simulink model "UnitTestDebug"  (R2018b)
settings: Solver=FixedStepAuto  StartTime=0.0  StopTime=500  FixedStep=fswParams.sample_time_s  RelTol=1e-3
undefined symbols (not defined in the file): DiscIntNeverNeededParam, fswParams, MEKF_lib, simParams, Triad, Triad_lib
libraries: aerolibutil x7, simulink x6, vrlib x4, sharedutil x3, sharedtransform x3, dspmathops x2, satelliteDynamics_lib x1
(part 1 of 2)
settings Model: SimulationMode=accelerator  Creator=satcave1  LastModifiedBy=kylle
settings OptimizationCC: EfficientMapNaN2IntZero=off
settings HardwareCC: TargetBitPerPointer=64  TargetBitPerSizeT=64  TargetBitPerPtrDiffT=64  TargetLongLongMode=on  TargetIntDivRoundTo=Zero  TargetEndianess=LittleEndian  TargetWordSize=64  TargetHWDeviceType=MATLAB Host  ProdEqTarget=off
settings CodeAppCC: MaxIdLength=128
settings GRTTargetCC: TargetLangStandard=C89/C90 (ANSI)  CombineOutputUpdateFcns=off  GRTInterface=on

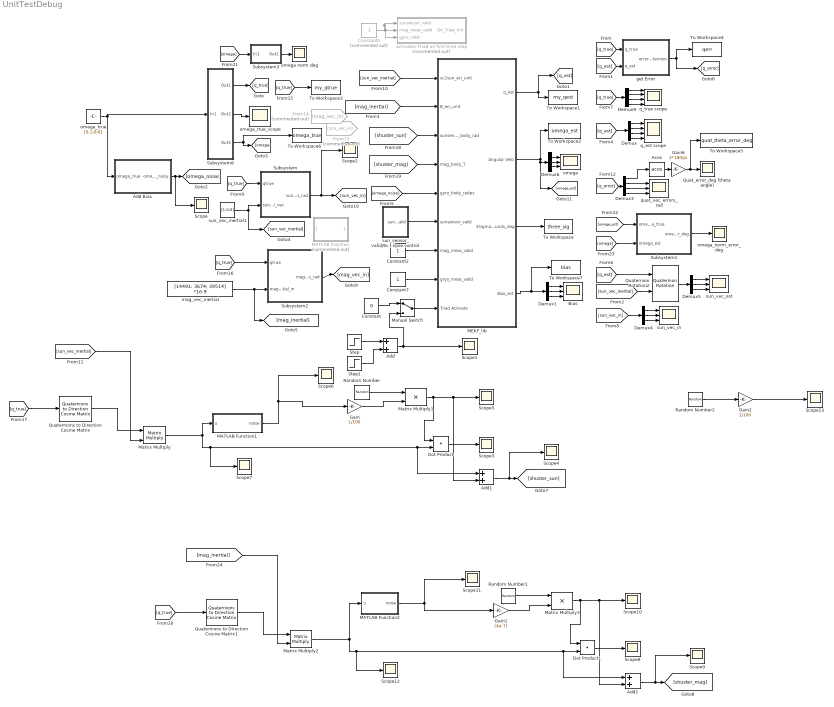
== system UnitTestDebug ==
  Acos : Trigonometry  Operator=acos
  Add : Sum
  Add Bias : Subsystem
  Add1 : Sum
  Add2 : Sum
  Bias : Scope  NumInputPorts=3
  Constant : Constant  Value=0
  Constant2 : Constant
  Constant5 : Constant  Commented=on
  Constant7 : Constant
  Demux : Demux
  Demux{1,4..6} (4 alike) : Demux  Outputs=3
  Demux3 : Demux
  Demux9 : Demux
  Dot Product : DotProduct  InputSameDT=on  OutDataTypeStr=Inherit: Inherit via internal rule
  Dot Product1 : DotProduct  InputSameDT=on  OutDataTypeStr=Inherit: Inherit via internal rule
  From13 : From  Commented=on  GotoTag=sun_vec_in
  From14 : From  Commented=on  GotoTag=mag_vec_in
  Gain : Gain  Gain=1/100
  Gain1 : Gain  Gain=(4e-7)
  Gain2 : Gain  Gain=1/100
  Gain6 : Gain  Gain=2*180/pi
  MATLAB Function : MATLAB Function  Commented=on  TreatAsAtomicUnit=on
  MATLAB Function1 : MATLAB Function  TreatAsAtomicUnit=on
  MATLAB Function2 : MATLAB Function  TreatAsAtomicUnit=on
  MEKF_lib : Subsystem  AncestorBlock=MEKF_lib/MEKF_lib
  Manual Switch : ManualSwitch
  Matrix Multiply : Product  Multiplication=Matrix(*)
  Matrix Multiply1 : Product
  Matrix Multiply2 : Product  Multiplication=Matrix(*)
  Matrix Multiply3 : Product
  Quat_error_deg (theta angle) : Scope
  Quaternion Rotation2 : aerolibutil/Quaternion Rotation
  Quaternions to Direction Cosine Matrix : sharedtransform/Quaternions to  Direction Cosine Matrix  aMode=aMode
      settings: SourceProductName=Aerospace Blockset  SourceProductBaseCode=AE
  Quaternions to Direction Cosine Matrix1 : sharedtransform/Quaternions to  Direction Cosine Matrix  aMode=aMode
      settings: SourceProductName=Aerospace Blockset  SourceProductBaseCode=AE
  Random Number : RandomNumber  Variance=[1;1;1]  SampleTime=0.1
  Random Number1 : RandomNumber  Variance=[1;1;1]  SampleTime=0.1
  Random Number2 : RandomNumber  Variance=[1;1;1]  SampleTime=0.1
  Scope{,1..13} (14 alike) : Scope
  Step : Step  Time=300  SampleTime=0
  Step1 : Step  Time=fswParams.sample_time_s+340  After=-1  SampleTime=0
  Subsystem : Subsystem
  Subsystem1 : Subsystem
  Subsystem2 : Subsystem
  Subsystem3 : Subsystem
  Subsystem8 : Subsystem
  To Workspace : ToWorkspace  VariableName=three_sig  SaveFormat=Structure With Time  SampleTime=-1
  To Workspace1 : ToWorkspace  VariableName=my_qest  SaveFormat=Structure With Time  SampleTime=-1
  To Workspace2 : ToWorkspace  VariableName=omega_est  SaveFormat=Structure  SampleTime=-1
  To Workspace3 : ToWorkspace  VariableName=my_qtrue  SaveFormat=Structure With Time  SampleTime=-1
  To Workspace4 : ToWorkspace  VariableName=qerr  SaveFormat=Structure With Time  SampleTime=-1
  To Workspace5 : ToWorkspace  VariableName=quat_theta_error_deg  SaveFormat=Structure With Time  SampleTime=-1
  To Workspace6 : ToWorkspace  VariableName=omega_true  SaveFormat=Structure  SampleTime=-1
  To Workspace7 : ToWorkspace  VariableName=bias  SaveFormat=Structure With Time  SampleTime=-1
  "activates Triad on first time step " : Subsystem  Commented=on
  get Error : Subsystem
  mag_vec_inertial : Constant  Value=[14491; 3674; 39514] *1e-9  VectorParams1D=off
  omega : Scope  NumInputPorts=3
  omega norm deg : Scope
  omega_norm_error_deg : Scope
  omega_true : Constant  Value=[0.1;0;0]  VectorParams1D=off
  omega_true_scope : Scope
  q_est scope : Scope  NumInputPorts=4
  "q_true scope " : Scope  NumInputPorts=4
  quat_vec_errors_rad : Scope  NumInputPorts=3
  sun_sensor_valid/Eclipse control : Subsystem
  sun_vec_est : Scope  NumInputPorts=3
  sun_vec_in : Scope  NumInputPorts=3
  sun_vec_inertial1 : Constant  Value=[1;0;0]  VectorParams1D=off
  wires:
  Demux/2 -> q_est scope/2
  Demux/3 -> q_est scope/3
  Demux/4 -> q_est scope/4
  Demux1/2 -> Bias/2
  Demux1/1 -> Bias/1
  Demux1/3 -> Bias/3
  Constant7/1 -> MEKF_lib/8(gryo_meas_valid)
  [sun_vec_inertial] -> MEKF_lib/1(sc2sun_eci_unit)
  [mag_inertial] -> MEKF_lib/2(B_eci_unit)
  MEKF_lib/3("3Sigma Bounds_deg ") -> To Workspace/1
  MEKF_lib/4(Bias_est) -> To Workspace7/1, Demux1/1
  MEKF_lib/1(q_est) -> To Workspace1/1, [q_est]
  [omega_noise] -> MEKF_lib/5(gyro_body_radps)
  Demux4/1 -> sun_vec_in/1
  Demux4/3 -> sun_vec_in/3
  Demux4/2 -> sun_vec_in/2
  [sun_vec_inertial] -> Quaternion Rotation2/2
  [q_est] -> Quaternion Rotation2/1
  Quaternion Rotation2/1 -> Demux5/1
  Demux5/1 -> sun_vec_est/1
  Demux5/2 -> sun_vec_est/2
  Demux6/1 -> omega/1
  Demux6/3 -> omega/3
  MEKF_lib/2("Angular Velo ") -> [omege_est], Demux6/1, To Workspace2/1
  Add/1 -> Manual Switch/2, Scope1/1
  Constant5/1 -> "activates Triad on first time step "/1(sunsensor_valid), "activates Triad on first time step "/3(gyro_valid), "activates Triad on first time step "/2(mag_meas_valid)
  Demux5/3 -> sun_vec_est/3
  Demux3/2 -> quat_vec_errors_rad/1
  Demux3/4 -> quat_vec_errors_rad/3
  [q_true] -> Demux9/1
  [q_true] -> get Error/1(q_true)
  [q_est] -> get Error/2(q_est)
  [sun_vec_in] -> Demux4/1
  [q_true] -> To Workspace3/1
  [q_est] -> Demux/1
  Demux/1 -> q_est scope/1
  Demux9/4 -> "q_true scope "/4
  Demux9/3 -> "q_true scope "/3
  Demux9/2 -> "q_true scope "/2
  Demux9/1 -> "q_true scope "/1
  Demux3/3 -> quat_vec_errors_rad/2
  get Error/1(error_quaternion) -> To Workspace4/1, [q_error]
  Constant2/1 -> MEKF_lib/7(mag_meas_valid)
  Demux3/1 -> Acos/1
  Acos/1 -> Gain6/1
  Gain6/1 -> To Workspace5/1, Quat_error_deg (theta angle)/1
  Subsystem8/1(Out1) -> [q_true]
  Subsystem8/2(Out2) -> omega_true_scope/1
  Subsystem8/3(Out5) -> [omega], To Workspace6/1
  [omege_est] -> Subsystem1/1(omega_true)
  [omega] -> Subsystem1/2(omega_est)
  Subsystem1/1(omega_norm_error_deg) -> omega_norm_error_deg/1
  [q_error] -> Demux3/1
  sun_sensor_valid/Eclipse control/1(sun_valid) -> MEKF_lib/6(sunsensor_valid)
  Demux6/2 -> omega/2
  Subsystem2/1(mag_body_meas_rad) -> [mag_vec_in]
  [q_true] -> Subsystem2/1(qtrue)
  mag_vec_inertial/1 -> [mag_inertial], Subsystem2/2(mag_inertial_in)
  [omega] -> Subsystem3/1(In1)
  Subsystem3/1(Out1) -> omega norm deg/1
  omega_true/1 -> Subsystem8/1(In1), Add Bias/1(omega_true)
  Add Bias/1(omega_noisy) -> Scope/1, [omega_noise]
  [q_true] -> Subsystem/1(qtrue)
  sun_vec_inertial1/1 -> [sun_vec_inertial], Subsystem/2(sun_inertial_vec)
  Subsystem/1(sun_vec_meas_rad) -> Scope2/1, [sun_vec_in]
  Step/1 -> Add/1
  Step1/1 -> Add/2
  Constant/1 -> Manual Switch/1
  Manual Switch/1 -> MEKF_lib/9(Triad Activate)
  [sun_vec_inertial] -> Matrix Multiply/2
  Quaternions to Direction Cosine Matrix/1 -> Matrix Multiply/1
  [q_true] -> Quaternions to Direction Cosine Matrix/1
  Matrix Multiply/1 -> MATLAB Function1/1(u), Scope7/1, Add1/1, Dot Product/2
  Dot Product/1 -> Scope3/1
  [shuster_sun] -> MEKF_lib/3(sunsensor_body_rad)
  Add1/1 -> Scope4/1, [shuster_sun]
  Random Number/1 -> Matrix Multiply1/1
  Matrix Multiply1/1 -> Dot Product/1, Add1/2, Scope5/1
  Gain/1 -> Matrix Multiply1/2
  MATLAB Function1/1(noise) -> Scope6/1, Gain/1
  Add2/1 -> Scope9/1, [shuster_mag]
  Matrix Multiply3/1 -> Dot Product1/1, Add2/2, Scope10/1
  Random Number1/1 -> Matrix Multiply3/1
  Quaternions to Direction Cosine Matrix1/1 -> Matrix Multiply2/1
  [mag_inertial] -> Matrix Multiply2/2
  [q_true] -> Quaternions to Direction Cosine Matrix1/1
  Gain1/1 -> Matrix Multiply3/2
  Matrix Multiply2/1 -> MATLAB Function2/1(u), Scope12/1, Add2/1, Dot Product1/2
  MATLAB Function2/1(noise) -> Gain1/1, Scope11/1
  Dot Product1/1 -> Scope8/1
  [shuster_mag] -> MEKF_lib/4(mag_body_T)
  Gain2/1 -> Scope13/1
  Random Number2/1 -> Gain2/1

== system UnitTestDebug/Add Bias ==
  note: concatenates the sensor measurements
      | into a 3 x N_gyro matrix
  omega_true : Inport
  Scope : Scope
  Terminator : Terminator
  Terminator1 : Terminator
  gyroscope_lib : Subsystem  mask{id_s=1}
      mask prompts: id_s "Choose the sensor ID"
      mask TypeOptions id_s: 1 | 2 | 3
      mask DialogControl DescTextVar Prompt: SOCi gyroscope model. The spacecraft has three Bosch BMI055 gyroscopes.
  omega_noisy : Outport
  wires:
  gyroscope_lib/2(bias_out) -> [bias_1]
  omega_true/1 -> gyroscope_lib/1(omega_in_radps)
  gyroscope_lib/1(omega_radps) -> [w_radps_1]
  [w_radps_1] -> omega_noisy/1
  gyroscope_lib/3(gyro_valid) -> [valid_1]
  [bias_1] -> Scope/1, Terminator/1
  [valid_1] -> Terminator1/1

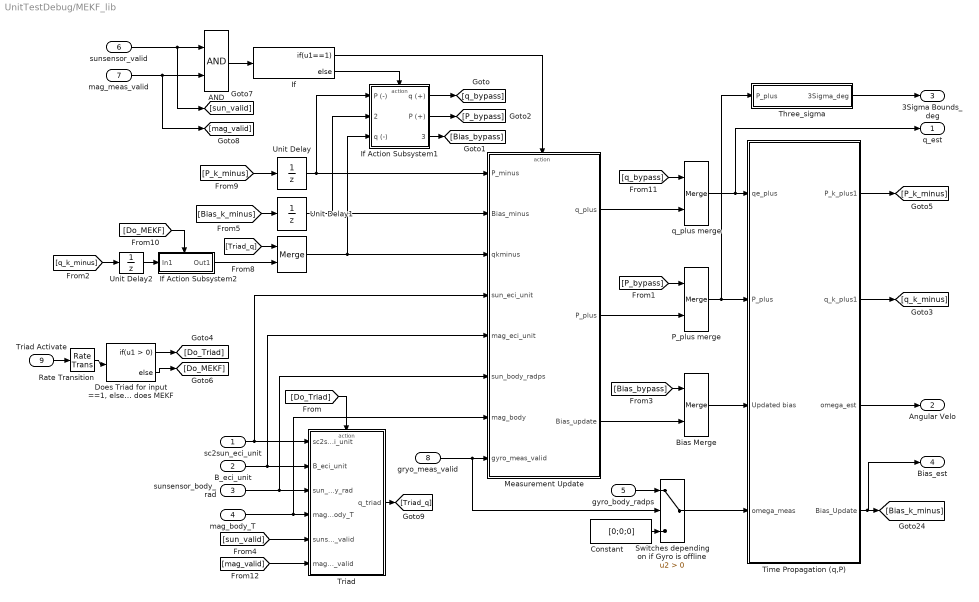
== system UnitTestDebug/MEKF_lib ==
  sc2sun_eci_unit : Inport
  B_eci_unit : Inport  Port=2
  sunsensor_body_rad : Inport  Port=3
  mag_body_T : Inport  Port=4
  gyro_body_radps : Inport  Port=5
  sunsensor_valid : Inport  Port=6
  mag_meas_valid : Inport  Port=7
  gryo_meas_valid : Inport  Port=8
  Triad Activate : Inport  Port=9
  " " : Merge
  AND : Logic  AllPortsSameDT=off  OutDataTypeStr=boolean
  Bias Merge : Merge
  Constant : Constant  Value=[0;0;0]
  "Does Triad for input ==1, else does MEKF" : If
  If : If  IfExpression=u1==1
  If Action Subsystem1 : Subsystem  TreatAsAtomicUnit=on
  If Action Subsystem2 : Subsystem  TreatAsAtomicUnit=on
  Measurement Update : Subsystem  TreatAsAtomicUnit=on
  P_plus merge : Merge
  Rate Transition : RateTransition  OutPortSampleTime=fswParams.sample_time_s
  "Switches depending on if Gyro is offline " : Switch  Criteria=u2 > Threshold
  Three_sigma : Subsystem
  Time Propagation (q,P) : Subsystem  AncestorBlock=MEKF_Library/Multiplicative Extended Kalman Filter/TIME PROPAGATION of Q_EST, COVARIANCE
  Triad : Subsystem  AncestorBlock=Triad_lib/Triad  TreatAsAtomicUnit=on
  Unit Delay : UnitDelay  InitialCondition=fswParams.estimation.ic.Pchol_init  SampleTime=fswParams.sample_time_s
  Unit Delay1 : UnitDelay  InitialCondition=fswParams.estimation.ic.Beta_init  SampleTime=fswParams.sample_time_s
  Unit Delay2 : UnitDelay  InitialCondition=fswParams.estimation.ic.quat_est_init  SampleTime=fswParams.sample_time_s
  q_plus merge : Merge
  q_est : Outport
  "Angular Velo " : Outport  Port=2
  "3Sigma Bounds_deg " : Outport  Port=3
  Bias_est : Outport  Port=4
  wires:
  AND/1 -> If/1
  mag_meas_valid/1 -> AND/2, [mag_valid]
  sunsensor_valid/1 -> AND/1, [sun_valid]
  "Does Triad for input ==1, else does MEKF"/2 -> [Do_MEKF]
  "Does Triad for input ==1, else does MEKF"/1 -> [Do_Triad]
  Triad Activate/1 -> Rate Transition/1
  Rate Transition/1 -> "Does Triad for input ==1, else does MEKF"/1
  Triad/1(q_triad) -> [Triad_q]
  [Do_Triad] -> Triad/Action
  If Action Subsystem2/1(Out1) -> " "/2
  [Triad_q] -> " "/1
  [q_k_minus] -> Unit Delay2/1
  Unit Delay2/1 -> If Action Subsystem2/1(In1)
  [Do_MEKF] -> If Action Subsystem2/Action
  sunsensor_body_rad/1 -> Triad/3(sun_body_rad), Measurement Update/6(sun_body_radps)
  mag_body_T/1 -> Triad/4(mag_body_T), Measurement Update/7(mag_body)
  [mag_valid] -> Triad/6(magsensor_valid)
  [sun_valid] -> Triad/5(sunsensor_valid)
  B_eci_unit/1 -> Triad/2(B_eci_unit), Measurement Update/5(mag_eci_unit)
  sc2sun_eci_unit/1 -> Triad/1(sc2sun_eci_unit), Measurement Update/4(sun_eci_unit)
  " "/1 -> If Action Subsystem1/3(q (-)), Measurement Update/3(qkminus)
  Unit Delay/1 -> Measurement Update/1(P_minus), If Action Subsystem1/1(P (-))
  Unit Delay1/1 -> Measurement Update/2(Bias_minus), If Action Subsystem1/2(Bias (-))
  Time Propagation (q,P)/2(q_k_plus1) -> [q_k_minus]
  Time Propagation (q,P)/1(P_k_plus1) -> [P_k_minus]
  If/1 -> Measurement Update/Action
  If/2 -> If Action Subsystem1/Action
  [Bias_k_minus] -> Unit Delay1/1
  [P_k_minus] -> Unit Delay/1
  Measurement Update/1(q_plus) -> q_plus merge/2
  Measurement Update/3(Bias_update) -> Bias Merge/2
  "Switches depending on if Gyro is offline "/1 -> Time Propagation (q,P)/4(omega_meas)
  If Action Subsystem1/1(q (+)) -> [q_bypass]
  [q_bypass] -> q_plus merge/1
  [Bias_bypass] -> Bias Merge/1
  If Action Subsystem1/2(P (+)) -> [P_bypass]
  If Action Subsystem1/3(Bias (+)) -> [Bias_bypass]
  Bias Merge/1 -> Time Propagation (q,P)/3(Updated bias)
  gryo_meas_valid/1 -> "Switches depending on if Gyro is offline "/2, Measurement Update/8(gyro_meas_valid)
  gyro_body_radps/1 -> "Switches depending on if Gyro is offline "/1
  Constant/1 -> "Switches depending on if Gyro is offline "/3
  P_plus merge/1 -> Time Propagation (q,P)/2(P_plus), Three_sigma/1(P_plus)
  [P_bypass] -> P_plus merge/1
  Measurement Update/2(P_plus) -> P_plus merge/2
  Time Propagation (q,P)/4(Bias_Update) -> [Bias_k_minus], Bias_est/1
  Three_sigma/1(3Sigma_deg) -> "3Sigma Bounds_deg "/1
  Time Propagation (q,P)/3(omega_est) -> "Angular Velo "/1
  q_plus merge/1 -> Time Propagation (q,P)/1(qe_plus), q_est/1

== system UnitTestDebug/Subsystem ==
  qtrue : Inport
  sun_inertial_vec : Inport  Port=2
  Add : Sum
  Add Gaussian Noise : Subsystem  Commented=on
  Dot Product : DotProduct  InputSameDT=on  OutDataTypeStr=Inherit: Inherit via internal rule
  From5 : From  Commented=on  GotoTag=sun_body
  Gain : Gain  Gain=1/1000
  Goto4 : Goto  Commented=on  GotoTag=sun_body
  MATLAB Function : MATLAB Function  TreatAsAtomicUnit=on
  Scope{,1..3} (4 alike) : Scope
  Subsystem6 : Subsystem
  sun_vec_meas_rad : Outport
  wires:
  Subsystem6/1(sun_vec_true_rad) -> Scope1/1, Dot Product/1, Add/1, MATLAB Function/1(v_input), Goto4/1
  From5/1 -> Add Gaussian Noise/1(sun_body_rad)
  sun_inertial_vec/1 -> Subsystem6/2(sun_inertial_vec)
  qtrue/1 -> Subsystem6/1(q_true)
  Gain/1 -> Add/2
  Add/1 -> Scope3/1, sun_vec_meas_rad/1
  MATLAB Function/1(v_perp) -> Scope2/1, Dot Product/2, Gain/1
  Dot Product/1 -> Scope/1

== system UnitTestDebug/Subsystem1 ==
  omega_true : Inport
  omega_est : Inport  Port=2
  Add4 : Sum  Inputs=-+
  Gain2 : Gain  Gain=180/pi
  Subsystem4 : Subsystem
  Subsystem5 : Subsystem
  omega_norm_error_deg : Outport
  wires:
  Add4/1 -> Gain2/1
  Subsystem5/1(Out1) -> Add4/2
  omega_true/1 -> Subsystem4/1(In1)
  Subsystem4/1(Out1) -> Add4/1
  Gain2/1 -> omega_norm_error_deg/1
  omega_est/1 -> Subsystem5/1(In1)

== system UnitTestDebug/Subsystem2 ==
  qtrue : Inport
  mag_inertial_in : Inport  Port=2
  Quaternion Rotation1 : aerolibutil/Quaternion Rotation
  Scope : Scope
  add Gaussian noise : Subsystem
  mag_body_meas_rad : Outport
  wires:
  qtrue/1 -> Quaternion Rotation1/1
  add Gaussian noise/1(maG_body_meas_rad) -> Scope/1, mag_body_meas_rad/1
  Quaternion Rotation1/1 -> [mag_body_true]
  [mag_body_true] -> add Gaussian noise/1(mag_body_true_rad)
  mag_inertial_in/1 -> Quaternion Rotation1/2

== system UnitTestDebug/Subsystem3 ==
  In1 : Inport
  Gain1 : Gain  Gain=180/pi
  norm_omega : Subsystem
  Out1 : Outport
  wires:
  norm_omega/1(Out1) -> Gain1/1
  Gain1/1 -> Out1/1
  In1/1 -> norm_omega/1(In1)

== system UnitTestDebug/Subsystem8 ==
  In1 : Inport
  Add3 : Sum  Inputs=+++
  Manual Switch1 : ManualSwitch
  Ramp : simulink/Sources/Ramp  slope=0.008  start=0  InitialOutput=0
  Ramp1 : simulink/Sources/Ramp  slope=-0.008  start=20  InitialOutput=0
  quat_propagation : satelliteDynamics_lib/satelliteDynamics_lib/quat_propagation  SystemSampleTime=-1
      link override Discrete-Time Integrator: InitialCondition=simParams.initialConditions.q0
  Out1 : Outport
  Out2 : Outport  Port=2
  Out5 : Outport  Port=3
  wires:
  Ramp/1 -> Add3/2
  Ramp1/1 -> Add3/3
  Manual Switch1/1 -> Out2/1, Out5/1, quat_propagation/1
  In1/1 -> Add3/1, Manual Switch1/1
  Add3/1 -> Manual Switch1/2
  quat_propagation/1 -> Out1/1

== system UnitTestDebug/activates Triad on first time step  ==
  sunsensor_valid : Inport
  mag_meas_valid : Inport  Port=2
  gyro_valid : Inport  Port=3
  AND : Logic  Inputs=3  IconShape=distinctive  AllPortsSameDT=off  OutDataTypeStr=boolean
  Compare To Constant : simulink/Logic and Bit Operations/Compare To Constant  relop===  const=1  OutDataTypeStr=boolean
  Memory : Memory
  OR : Logic  Operator=OR  AllPortsSameDT=off  OutDataTypeStr=boolean
  Do_Triad_Init : Outport
  wires:
  mag_meas_valid/1 -> AND/2
  Compare To Constant/1 -> OR/2
  OR/1 -> Do_Triad_Init/1, Memory/1
  Memory/1 -> OR/1
  AND/1 -> Compare To Constant/1
  sunsensor_valid/1 -> AND/1
  gyro_valid/1 -> AND/3

== system UnitTestDebug/get Error ==
  q_true : Inport
  q_est : Inport  Port=2
  Quaternion Conjugate : aerolibutil/Quaternion Conjugate
      settings: SourceProductName=Aerospace Blockset  SourceProductBaseCode=AE
  Quaternion Multiplication : aerolibutil/Quaternion Multiplication
  error_quaternion : Outport
  wires:
  Quaternion Conjugate/1 -> Quaternion Multiplication/1
  Quaternion Multiplication/1 -> error_quaternion/1
  q_true/1 -> Quaternion Conjugate/1
  q_est/1 -> Quaternion Multiplication/2

== system UnitTestDebug/sun_sensor_valid//Eclipse control ==
  Add2 : Sum  Inputs=+++
  Constant6 : Constant
  Eclipse_end : Step  Time=3700.0333  SampleTime=0
  Eclipse_time : Step  Time=1900  After=-1  SampleTime=0
  Manual Switch : ManualSwitch
  Scope3 : Scope
  Step : Step  Time=0  SampleTime=0
  sun_valid : Outport
  wires:
  Add2/1 -> Manual Switch/2, Scope3/1
  Eclipse_time/1 -> Add2/2
  Step/1 -> Add2/1
  Constant6/1 -> Manual Switch/1
  Eclipse_end/1 -> Add2/3
  Manual Switch/1 -> sun_valid/1

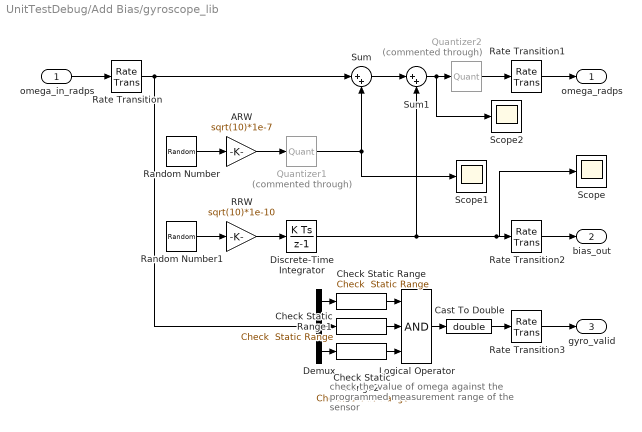
== system UnitTestDebug/Add Bias/gyroscope_lib ==
  note: check the value of omega against
      | the programmed measurement range
      | of the sensor
  omega_in_radps : Inport
  ARW : Gain  Gain=sqrt(10)*1e-7
  Cast To Double : DataTypeConversion  OutDataTypeStr=double
  Check Static Range : simulink/Model Verification/Check  Static Range  Description=simParams.sensors.gyro.w_min(id_s) <= u <= simParams.sensors.gyro.w_max(id_s)  max=simParams.sensors.gyro.w_max(id_s)  max_included=on  min=simParams.sensors.gyro.w_min(id_s)  min_included=on  enabled=on  stopWhenAssertionFail=off  export=on  icon=graphic
      settings: SourceProductName=Simulink  SourceProductBaseCode=SL
  Check Static Range1 : simulink/Model Verification/Check  Static Range  Description=simParams.sensors.gyro.w_min(id_s) <= u <= simParams.sensors.gyro.w_max(id_s)  max=simParams.sensors.gyro.w_max(id_s)  max_included=on  min=simParams.sensors.gyro.w_min(id_s)  min_included=on  enabled=on  stopWhenAssertionFail=off  export=on  icon=graphic
      settings: SourceProductName=Simulink  SourceProductBaseCode=SL
  Check Static Range2 : simulink/Model Verification/Check  Static Range  Description=simParams.sensors.gyro.w_min(id_s) <= u <= simParams.sensors.gyro.w_max(id_s)  max=simParams.sensors.gyro.w_max(id_s)  max_included=on  min=simParams.sensors.gyro.w_min(id_s)  min_included=on  enabled=on  stopWhenAssertionFail=off  export=on  icon=graphic
      settings: SourceProductName=Simulink  SourceProductBaseCode=SL
  Demux : Demux  Outputs=3
  Discrete-Time Integrator : DiscreteIntegrator  InitialCondition=simParams.sensors.gyro.bias_init(id_s)  SampleTime=-1  ICPrevOutput=DiscIntNeverNeededParam  ICPrevScaledInput=DiscIntNeverNeededParam
  Logical Operator : Logic  Inputs=3  AllPortsSameDT=off  OutDataTypeStr=boolean
  Quantizer1 : Quantizer  Commented=through  QuantizationInterval=simParams.sensors.gyro.resolution(id_s)
  Quantizer2 : Quantizer  Commented=through  QuantizationInterval=simParams.sensors.gyro.resolution(id_s)
  RRW : Gain  Gain=sqrt(10)*1e-10
  Random Number : RandomNumber  Mean=[0 0 0]  Variance=[1 1 1]  Seed=simParams.sensors.gyro.seed_arw(:,id_s)  SampleTime=simParams.sensors.gyro.sample_time_s
  Random Number1 : RandomNumber  Mean=[0 0 0]  Variance=[1 1 1]  Seed=simParams.sensors.gyro.seed_rrw(:,id_s)  SampleTime=simParams.sensors.gyro.sample_time_s
  Rate Transition : RateTransition  InitialCondition=simParams.initialConditions.w0  OutPortSampleTime=simParams.sensors.gyro.sample_time_s
  Rate Transition1 : RateTransition  InitialCondition=simParams.initialConditions.w0
  Rate Transition2 : RateTransition  InitialCondition=simParams.sensors.gyro.bias_init(id_s)
  Rate Transition3 : RateTransition  InitialCondition=1
  Scope : Scope
  Scope1 : Scope
  Scope2 : Scope
  Sum : Sum  Inputs=|++
  Sum1 : Sum  Inputs=|++
  omega_radps : Outport
  bias_out : Outport  Port=2
  gyro_valid : Outport  Port=3
  wires:
  Logical Operator/1 -> Cast To Double/1
  Check Static Range2/1 -> Logical Operator/3
  Check Static Range/1 -> Logical Operator/1
  Check Static Range1/1 -> Logical Operator/2
  Demux/1 -> Check Static Range/1
  Demux/2 -> Check Static Range1/1
  Demux/3 -> Check Static Range2/1
  Rate Transition3/1 -> gyro_valid/1
  Rate Transition2/1 -> bias_out/1
  Rate Transition1/1 -> omega_radps/1
  Rate Transition/1 -> Sum/1, Demux/1
  Quantizer2/1 -> Rate Transition1/1
  Sum1/1 -> Scope2/1, Quantizer2/1
  Quantizer1/1 -> Sum/2, Scope1/1
  Discrete-Time Integrator/1 -> Sum1/2, Scope/1, Rate Transition2/1
  Cast To Double/1 -> Rate Transition3/1
  RRW/1 -> Discrete-Time Integrator/1
  Sum/1 -> Sum1/1
  omega_in_radps/1 -> Rate Transition/1
  ARW/1 -> Quantizer1/1
  Random Number1/1 -> RRW/1
  Random Number/1 -> ARW/1

== system UnitTestDebug/MEKF_lib/If Action Subsystem1 ==
  P (-) : Inport
  Bias (-) : Inport  Port=2
  q (-) : Inport  Port=3
  Action Port : ActionPort  ActionType=else
  q (+) : Outport
  P (+) : Outport  Port=2
  Bias (+) : Outport  Port=3
  wires:
  P (-)/1 -> P (+)/1
  Bias (-)/1 -> Bias (+)/1
  q (-)/1 -> q (+)/1

== system UnitTestDebug/MEKF_lib/If Action Subsystem2 ==
  In1 : Inport
  Action Port : ActionPort  ActionType=else
  Out1 : Outport
  wires:
  In1/1 -> Out1/1

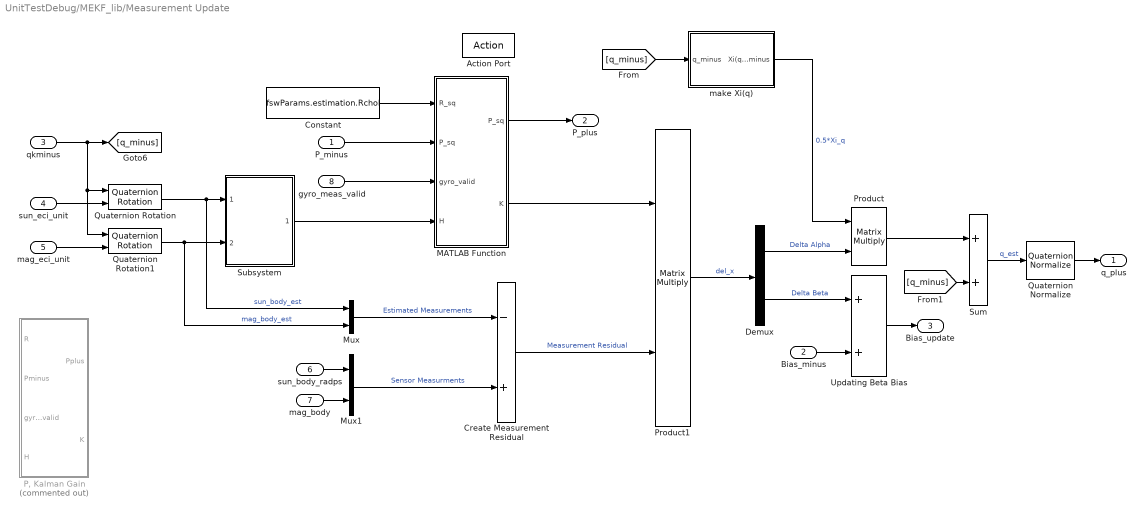
== system UnitTestDebug/MEKF_lib/Measurement Update ==
  P_minus : Inport
  Bias_minus : Inport  Port=2
  qkminus : Inport  Port=3
  sun_eci_unit : Inport  Port=4
  mag_eci_unit : Inport  Port=5
  sun_body_radps : Inport  Port=6
  mag_body : Inport  Port=7
  gyro_meas_valid : Inport  Port=8
  Action Port : ActionPort  ActionType=then
  Constant : Constant  Value=fswParams.estimation.Rchol  VectorParams1D=off
  Create Measurement Residual : Sum  Inputs=-+
  Demux : Demux  Outputs=2
  MATLAB Function : MATLAB Function  TreatAsAtomicUnit=on
  Mux : Mux  Inputs=2
  Mux1 : Mux  Inputs=2
  "P, Kalman Gain" : MATLAB Function  Commented=on  TreatAsAtomicUnit=on
  Product : Product  Inputs=**  Multiplication=Matrix(*)
  Product1 : Product  Multiplication=Matrix(*)
  Quaternion Normalize : sharedutil/Quaternion Normalize  aMode=aMode
      settings: SourceProductName=Aerospace Blockset  SourceProductBaseCode=AE
  Quaternion Rotation : aerolibutil/Quaternion Rotation
  Quaternion Rotation1 : aerolibutil/Quaternion Rotation
  Subsystem : Subsystem
  Sum : Sum
  "Updating Beta Bias " : Sum
  make Xi(q) : Subsystem
  q_plus : Outport
  P_plus : Outport  Port=2
  Bias_update : Outport  Port=3
  wires:
  [q_minus] -> make Xi(q)/1(q_minus)
  qkminus/1 -> [q_minus], Quaternion Rotation/1, Quaternion Rotation1/1
  Quaternion Rotation/1 -> Mux/1, Subsystem/1(sun_body_hat)  "sun_body_est"
  Quaternion Rotation1/1 -> Mux/2, Subsystem/2(mag_body_hat)  "mag_body_est"
  mag_eci_unit/1 -> Quaternion Rotation1/2
  sun_eci_unit/1 -> Quaternion Rotation/2
  "Updating Beta Bias "/1 -> Bias_update/1
  sun_body_radps/1 -> Mux1/1
  mag_body/1 -> Mux1/2
  Create Measurement Residual/1 -> Product1/2  "Measurement Residual"
  Quaternion Normalize/1 -> q_plus/1
  make Xi(q)/1(Xi(q)_minus) -> Product/1  "0.5*Xi_q"
  Demux/1 -> Product/2  "Delta Alpha"
  Product1/1 -> Demux/1  "del_x"
  Product/1 -> Sum/1
  Sum/1 -> Quaternion Normalize/1  "q_est"
  Bias_minus/1 -> "Updating Beta Bias "/2
  Mux/1 -> Create Measurement Residual/1  "Estimated Measurements"
  Demux/2 -> "Updating Beta Bias "/1  "Delta Beta"
  Mux1/1 -> Create Measurement Residual/2  "Sensor Measurments"
  [q_minus] -> Sum/2
  Constant/1 -> MATLAB Function/1(R_sq)
  P_minus/1 -> MATLAB Function/2("P_sq ")
  gyro_meas_valid/1 -> MATLAB Function/3(gyro_valid)
  Subsystem/1(H_matrix) -> MATLAB Function/4(H)
  MATLAB Function/1(P_sq) -> P_plus/1
  MATLAB Function/2(K) -> Product1/1

== system UnitTestDebug/MEKF_lib/Three_sigma ==
  P_plus : Inport
  Abs : Abs
  Demux : Demux  Outputs=2
  Extract Diagonal : S-Function  AncestorBlock=dspmtrx3/Extract Diagonal  FunctionName=sdspdiag2  Parameters=mode  SFunctionDeploymentMode=off  EnableBusSupport=off  mask(Extract Diagonal){}
      mask help: Extract the main diagonal of a full matrix.
      mask init:
      | mode = 2;
      | x = [.58 .87 NaN 0.12 0.45 0.45 0.12 0.12 NaN 0.525 0.525 0.475 0.475 0.525 0.525 0.565 0.525 ];
      | y = [ 0.8 0.2 NaN 0.2 0.2 0.8 0.8 0.2 NaN 0.435 0.475 0.475 0.525 0.525 0.565 0.5 0.435 ];
      mask Help: eval('blocksethelp');
      mask Display:
      | plot(x,y);
      | port_label('input',1,'A');
      | port_label('output',1,'D');
  Multiply : Gain  Gain=3*180/pi
  Terminator : Terminator
  3Sigma_deg : Outport
  wires:
  Demux/2 -> Terminator/1
  Demux/1 -> Abs/1
  Extract Diagonal/1 -> Demux/1
  Abs/1 -> Multiply/1
  P_plus/1 -> Extract Diagonal/1
  Multiply/1 -> 3Sigma_deg/1

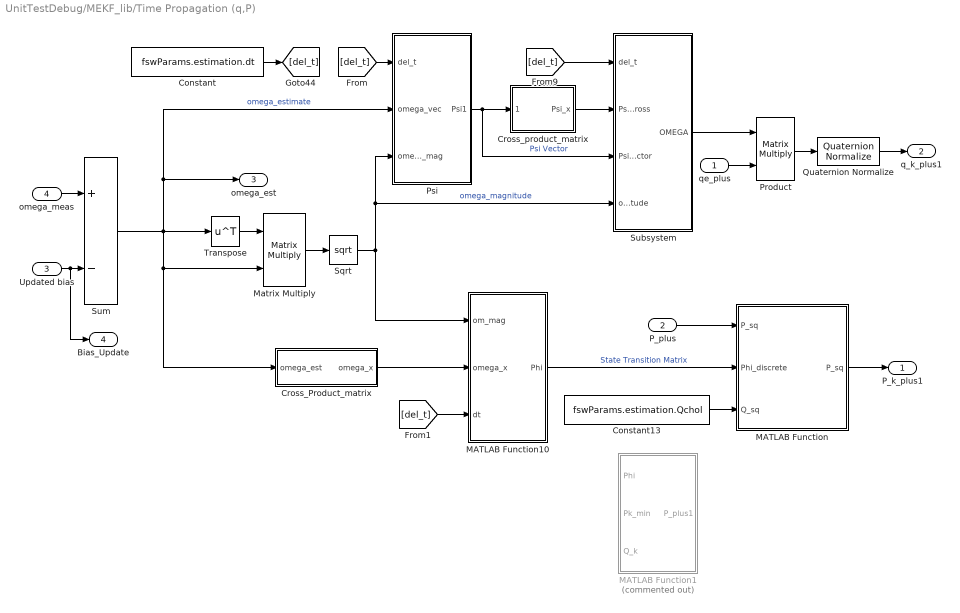
== system UnitTestDebug/MEKF_lib/Time Propagation (q,P) ==
  qe_plus : Inport
  P_plus : Inport  Port=2
  Updated bias : Inport  Port=3
  omega_meas : Inport  Port=4
  Constant : Constant  Value=fswParams.estimation.dt
  Constant13 : Constant  Value=fswParams.estimation.Qchol  VectorParams1D=off
  Cross_Product_matrix : Subsystem
  Cross_product_matrix : Subsystem
  MATLAB Function : MATLAB Function  TreatAsAtomicUnit=on
  MATLAB Function1 : MATLAB Function  Commented=on  TreatAsAtomicUnit=on
  MATLAB Function10 : MATLAB Function  TreatAsAtomicUnit=on
  Matrix Multiply : Product  Multiplication=Matrix(*)
  Product : Product  Multiplication=Matrix(*)
  Psi : Subsystem
  Quaternion Normalize : sharedutil/Quaternion Normalize  aMode=aMode
      settings: SourceProductName=Aerospace Blockset  SourceProductBaseCode=AE
  Sqrt : Sqrt  SaturateOnIntegerOverflow=on
  Subsystem : Subsystem
  Sum : Sum  Inputs=+-
  Transpose : Math  Operator=transpose  SaturateOnIntegerOverflow=on
  P_k_plus1 : Outport
  q_k_plus1 : Outport  Port=2
  omega_est : Outport  Port=3
  Bias_Update : Outport  Port=4
  wires:
  Subsystem/1(OMEGA) -> Product/1
  Cross_product_matrix/1(Psi_x) -> Subsystem/2(Psi_cross)
  Psi/1(Psi1) -> Cross_product_matrix/1(Psi_vec), Subsystem/3(Psi_vector)  "Psi Vector"
  [del_t] -> Subsystem/1(del_t)
  Cross_Product_matrix/1(omega_x) -> MATLAB Function10/2(omega_x)
  Sqrt/1 -> Subsystem/4(omega_magnitude), Psi/3(omega_mag), MATLAB Function10/1(om_mag)  "omega_magnitude"
  Updated bias/1 -> Sum/2, Bias_Update/1
  Transpose/1 -> Matrix Multiply/1
  Matrix Multiply/1 -> Sqrt/1
  Constant/1 -> [del_t]
  Sum/1 -> Transpose/1, Psi/2(omega_vec), omega_est/1, Matrix Multiply/2, Cross_Product_matrix/1(omega_est)  "omega_estimate"
  [del_t] -> Psi/1(del_t)
  qe_plus/1 -> Product/2
  [del_t] -> MATLAB Function10/3(dt)
  Product/1 -> Quaternion Normalize/1
  omega_meas/1 -> Sum/1
  Quaternion Normalize/1 -> q_k_plus1/1
  Constant13/1 -> MATLAB Function/3(Q_sq)
  P_plus/1 -> MATLAB Function/1("P_sq ")
  MATLAB Function10/1(Phi) -> MATLAB Function/2(Phi_discrete)  "State Transition Matrix"
  MATLAB Function/1(P_sq) -> P_k_plus1/1

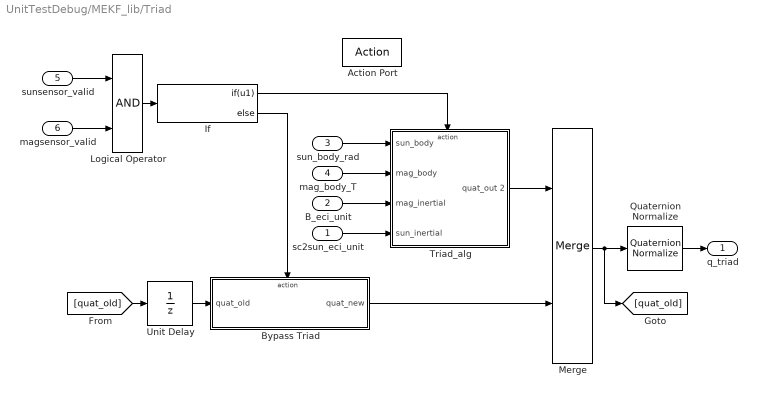
== system UnitTestDebug/MEKF_lib/Triad ==
  sc2sun_eci_unit : Inport
  B_eci_unit : Inport  Port=2
  sun_body_rad : Inport  Port=3
  mag_body_T : Inport  Port=4
  sunsensor_valid : Inport  Port=5
  magsensor_valid : Inport  Port=6
  Action Port : ActionPort  ActionType=then
  Bypass Triad : Subsystem  TreatAsAtomicUnit=on
  If : If  IfExpression=u1
  Logical Operator : Logic  AllPortsSameDT=off  OutDataTypeStr=boolean
  Merge : Merge
  Quaternion Normalize : sharedutil/Quaternion Normalize  aMode=aMode
      settings: SourceProductName=Aerospace Blockset  SourceProductBaseCode=AE
  Triad_alg : Subsystem  TreatAsAtomicUnit=on
  Unit Delay : UnitDelay  InitialCondition=fswParams.estimation.ic.quat_est_init  SampleTime=fswParams.sample_time_s
  q_triad : Outport
  wires:
  sc2sun_eci_unit/1 -> Triad_alg/4(sun_inertial)
  Unit Delay/1 -> Bypass Triad/1(quat_old)
  [quat_old] -> Unit Delay/1
  B_eci_unit/1 -> Triad_alg/3("mag_inertial ")
  sun_body_rad/1 -> Triad_alg/1(sun_body)
  mag_body_T/1 -> Triad_alg/2(mag_body)
  magsensor_valid/1 -> Logical Operator/2
  sunsensor_valid/1 -> Logical Operator/1
  Logical Operator/1 -> If/1
  Bypass Triad/1(quat_new) -> Merge/2
  Triad_alg/1(quat_out 2) -> Merge/1
  If/2 -> Bypass Triad/Action
  If/1 -> Triad_alg/Action
  Quaternion Normalize/1 -> q_triad/1
  Merge/1 -> [quat_old], Quaternion Normalize/1

== system UnitTestDebug/Subsystem/Add Gaussian Noise ==
  sun_body_rad : Inport
  Add : Sum
  Scope : Scope
  std deviation of sun sensor : Gain  Gain=5e-6
  sun noise : RandomNumber  Variance=[1;1;1]  SampleTime=fswParams.sample_time_s  VectorParams1D=off
  sun_meas_body_rad : Outport
  wires:
  sun noise/1 -> std deviation of sun sensor/1
  std deviation of sun sensor/1 -> Scope/1, Add/1
  Add/1 -> sun_meas_body_rad/1
  sun_body_rad/1 -> Add/2

== system UnitTestDebug/Subsystem/Subsystem6 ==
  q_true : Inport
  sun_inertial_vec : Inport  Port=2
  Quaternion Rotation : aerolibutil/Quaternion Rotation
  To Workspace6 : ToWorkspace  VariableName=sun_body_true  SaveFormat=Timeseries  SampleTime=-1
  sun_vec_true_rad : Outport
  wires:
  sun_inertial_vec/1 -> Quaternion Rotation/2
  q_true/1 -> Quaternion Rotation/1
  Quaternion Rotation/1 -> To Workspace6/1, sun_vec_true_rad/1

== system UnitTestDebug/Subsystem1/Subsystem4 ==
  In1 : Inport
  Matrix Multiply : Product  Multiplication=Matrix(*)
  Sqrt : Sqrt  SaturateOnIntegerOverflow=on
  Transpose : Math  Operator=transpose  SaturateOnIntegerOverflow=on
  Out1 : Outport
  wires:
  In1/1 -> Matrix Multiply/2, Transpose/1
  Transpose/1 -> Matrix Multiply/1
  Matrix Multiply/1 -> Sqrt/1
  Sqrt/1 -> Out1/1

== system UnitTestDebug/Subsystem1/Subsystem5 ==
  In1 : Inport
  Matrix Multiply : Product  Multiplication=Matrix(*)
  Sqrt : Sqrt  SaturateOnIntegerOverflow=on
  Transpose : Math  Operator=transpose  SaturateOnIntegerOverflow=on
  Out1 : Outport
  wires:
  In1/1 -> Matrix Multiply/2, Transpose/1
  Transpose/1 -> Matrix Multiply/1
  Matrix Multiply/1 -> Sqrt/1
  Sqrt/1 -> Out1/1

== system UnitTestDebug/Subsystem2/add Gaussian noise ==
  mag_body_true_rad : Inport
  Add1 : Sum
  mag noise : RandomNumber  Variance=[1;1;1]  SampleTime=fswParams.sample_time_s  VectorParams1D=off
  std deviation of mag sensor : Gain  Gain=2e-9
  maG_body_meas_rad : Outport
  wires:
  mag_body_true_rad/1 -> Add1/2
  std deviation of mag sensor/1 -> Add1/1
  mag noise/1 -> std deviation of mag sensor/1
  Add1/1 -> maG_body_meas_rad/1

== system UnitTestDebug/Subsystem3/norm_omega ==
  In1 : Inport
  Matrix Multiply : Product  Multiplication=Matrix(*)
  Sqrt : Sqrt  SaturateOnIntegerOverflow=on
  Transpose : Math  Operator=transpose  SaturateOnIntegerOverflow=on
  Out1 : Outport
  wires:
  In1/1 -> Matrix Multiply/2, Transpose/1
  Transpose/1 -> Matrix Multiply/1
  Matrix Multiply/1 -> Sqrt/1
  Sqrt/1 -> Out1/1

== system UnitTestDebug/MEKF_lib/Measurement Update/Subsystem ==
  sun_body_hat : Inport
  mag_body_hat : Inport  Port=2
  Constant1 : Constant  Value=zeros(3,3)  VectorParams1D=off
  Constant2 : Constant  Value=zeros(3,3)  VectorParams1D=off
  Cross_product_matrix2 : Subsystem  AncestorBlock=MEKF_lib/MEKF_lib/Measurement Update/Cross_product_matrix
  Cross_product_matrix3 : Subsystem  AncestorBlock=MEKF_lib/MEKF_lib/Measurement Update/Cross_product_matrix1
  Horizontal Matrix Concatenate : Concatenate  Mode=Multidimensional array
  Horizontal Matrix Concatenate1 : Concatenate  Mode=Multidimensional array
  Vertical Matrix Concatenate : Concatenate  Mode=Multidimensional array  ConcatenateDimension=2
  H_matrix : Outport
  wires:
  Constant1/1 -> Horizontal Matrix Concatenate1/2
  Constant2/1 -> Horizontal Matrix Concatenate1/1
  Cross_product_matrix3/1(mag_body_x) -> Horizontal Matrix Concatenate/2
  Horizontal Matrix Concatenate/1 -> Vertical Matrix Concatenate/1
  Horizontal Matrix Concatenate1/1 -> Vertical Matrix Concatenate/2
  sun_body_hat/1 -> Cross_product_matrix2/1(sun_body_hat)
  Cross_product_matrix2/1(sun_body_x) -> Horizontal Matrix Concatenate/1
  mag_body_hat/1 -> Cross_product_matrix3/1(mag_body_hat)
  Vertical Matrix Concatenate/1 -> H_matrix/1

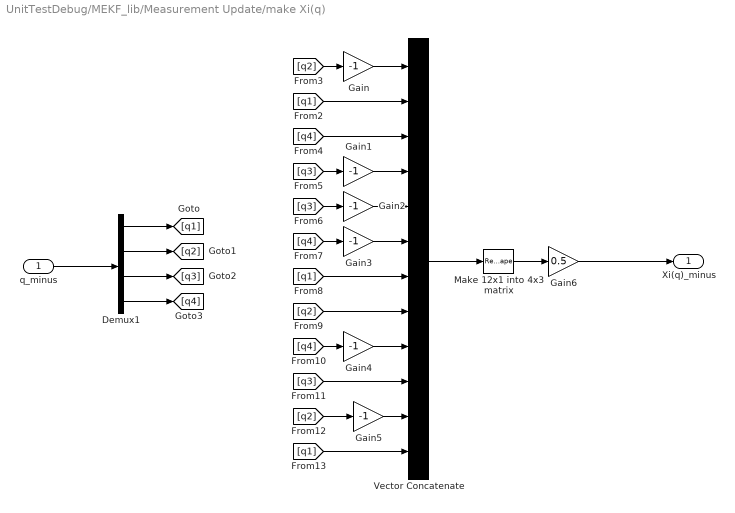
== system UnitTestDebug/MEKF_lib/Measurement Update/make Xi(q) ==
  q_minus : Inport
  Demux1 : Demux
  Gain{,1..5} (6 alike) : Gain  Gain=-1
  Gain6 : Gain  Gain=0.5
  Make 12x1 into 4x3 matrix : Reshape  OutputDimensionality=Customize  OutputDimensions=[4,3]
  Vector Concatenate : Concatenate  NumInputs=12
  Xi(q)_minus : Outport
  wires:
  Vector Concatenate/1 -> Make 12x1 into 4x3 matrix/1
  [q3] -> Gain2/1
  Gain3/1 -> Vector Concatenate/6
  [q1] -> Vector Concatenate/2
  Make 12x1 into 4x3 matrix/1 -> Gain6/1
  [q3] -> Gain1/1
  [q4] -> Gain3/1
  [q2] -> Gain/1
  [q3] -> Vector Concatenate/10
  Gain2/1 -> Vector Concatenate/5
  Gain1/1 -> Vector Concatenate/4
  Demux1/2 -> [q2]
  [q2] -> Vector Concatenate/8
  Demux1/1 -> [q1]
  Gain4/1 -> Vector Concatenate/9
  Demux1/3 -> [q3]
  [q4] -> Vector Concatenate/3
  [q1] -> Vector Concatenate/12
  Gain/1 -> Vector Concatenate/1
  [q2] -> Gain5/1
  [q4] -> Gain4/1
  Gain5/1 -> Vector Concatenate/11
  [q1] -> Vector Concatenate/7
  Demux1/4 -> [q4]
  q_minus/1 -> Demux1/1
  Gain6/1 -> Xi(q)_minus/1

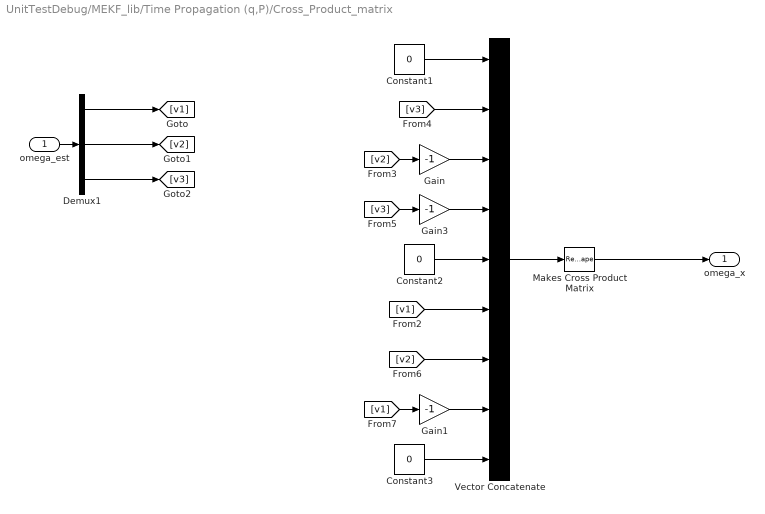
== system UnitTestDebug/MEKF_lib/Time Propagation (q,P)/Cross_Product_matrix ==
  omega_est : Inport
  Constant1 : Constant  Value=0
  Constant2 : Constant  Value=0
  Constant3 : Constant  Value=0
  Demux1 : Demux  Outputs=3
  Gain : Gain  Gain=-1
  Gain1 : Gain  Gain=-1
  Gain3 : Gain  Gain=-1
  Makes Cross Product Matrix : Reshape  OutputDimensionality=Customize  OutputDimensions=[3,3]
  Vector Concatenate : Concatenate  NumInputs=9
  omega_x : Outport
  wires:
  Gain1/1 -> Vector Concatenate/8
  Gain3/1 -> Vector Concatenate/4
  Gain/1 -> Vector Concatenate/3
  [v2] -> Gain/1
  [v3] -> Gain3/1
  Makes Cross Product Matrix/1 -> omega_x/1
  Constant2/1 -> Vector Concatenate/5
  Constant1/1 -> Vector Concatenate/1
  [v3] -> Vector Concatenate/2
  [v1] -> Gain1/1
  omega_est/1 -> Demux1/1
  [v1] -> Vector Concatenate/6
  Constant3/1 -> Vector Concatenate/9
  [v2] -> Vector Concatenate/7
  Demux1/3 -> [v3]
  Demux1/1 -> [v1]
  Demux1/2 -> [v2]
  Vector Concatenate/1 -> Makes Cross Product Matrix/1

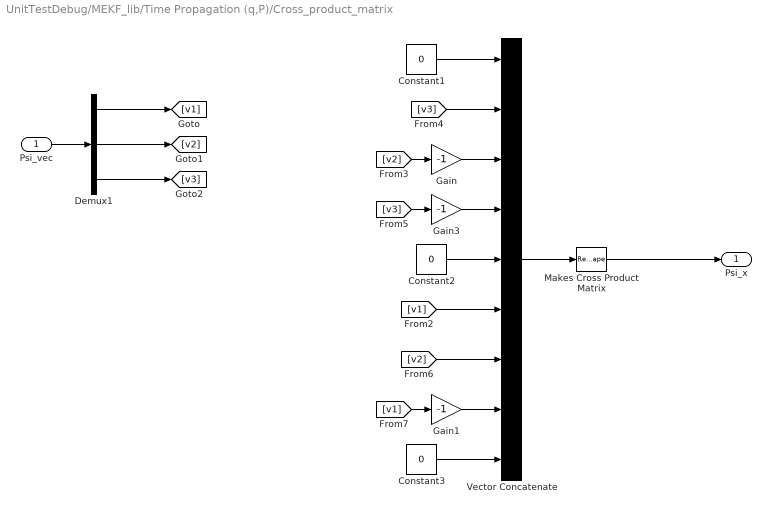
== system UnitTestDebug/MEKF_lib/Time Propagation (q,P)/Cross_product_matrix ==
  Psi_vec : Inport
  Constant1 : Constant  Value=0
  Constant2 : Constant  Value=0
  Constant3 : Constant  Value=0
  Demux1 : Demux  Outputs=3
  Gain : Gain  Gain=-1
  Gain1 : Gain  Gain=-1
  Gain3 : Gain  Gain=-1
  Makes Cross Product Matrix : Reshape  OutputDimensionality=Customize  OutputDimensions=[3,3]
  Vector Concatenate : Concatenate  NumInputs=9
  Psi_x : Outport
  wires:
  Demux1/1 -> [v1]
  [v1] -> Gain1/1
  Gain3/1 -> Vector Concatenate/4
  Constant2/1 -> Vector Concatenate/5
  [v1] -> Vector Concatenate/6
  [v2] -> Vector Concatenate/7
  Constant1/1 -> Vector Concatenate/1
  [v3] -> Vector Concatenate/2
  Demux1/2 -> [v2]
  Vector Concatenate/1 -> Makes Cross Product Matrix/1
  Gain1/1 -> Vector Concatenate/8
  Gain/1 -> Vector Concatenate/3
  Psi_vec/1 -> Demux1/1
  Makes Cross Product Matrix/1 -> Psi_x/1
  Demux1/3 -> [v3]
  [v2] -> Gain/1
  [v3] -> Gain3/1
  Constant3/1 -> Vector Concatenate/9

== system UnitTestDebug/MEKF_lib/Time Propagation (q,P)/Psi ==
  del_t : Inport
  omega_vec : Inport  Port=2
  omega_mag : Inport  Port=3
  If : If  IfExpression=u1<1e-10
  If Action Subsystem : Subsystem  TreatAsAtomicUnit=on
  If Action Subsystem1 : Subsystem  TreatAsAtomicUnit=on
  Merge : Merge
  Psi1 : Outport
  wires:
  omega_mag/1 -> If/1, If Action Subsystem/3(omega_mag)
  del_t/1 -> If Action Subsystem/1(del_t)
  omega_vec/1 -> If Action Subsystem/2(omega_vec)
  Merge/1 -> Psi1/1
  If Action Subsystem1/1(Psi_zero) -> Merge/1
  If/1 -> If Action Subsystem1/Action
  If Action Subsystem/1(Psi) -> Merge/2
  If/2 -> If Action Subsystem/Action

== system UnitTestDebug/MEKF_lib/Time Propagation (q,P)/Subsystem ==
  del_t : Inport
  Psi_cross : Inport  Port=2
  Psi_vector : Inport  Port=3
  omega_magnitude : Inport  Port=4
  Add1 : Sum  Inputs=+-
  Constant : Constant  Value=0.5
  Cos : Trigonometry  Operator=cos
  Gain : Gain  Gain=-1
  Identity Matrix : S-Function  AncestorBlock=dspmtrx3/Identity Matrix  FunctionName=sdspeye  Parameters=Inherit,N,Ts,isCustomFloat,fxpIsSigned,dTypeID,fxpWordLength,fxpFracLength,1  SFunctionDeploymentMode=off  EnableBusSupport=off  mask(Identity Matrix){Inherit=off, N=3, Ts=1, additionalParams=off, allowOverrides=on, dataType=double, isSigned=on, wordLen=16, udDataType=sfix(16), fracBitsMode=Best precision, numFracBits=15, OutDataTypeStr=double, LastOutDataTypeStr=double}
      mask prompts: Inherit "Inherit output port attributes from input port"; N "Matrix size:"; Ts "Sample time:"; additionalParams "------- Show additional parameters --------"; allowOverrides "Allow overrides by DSP Fixed-Point Attributes blocks"; dataType "Output data type:"; isSigned "Signed"; wordLen "Word length:"; udDataType "User-defined data type (e.g. sfix(16), float('single')):"; fracBitsMode "Set fraction length in output to:"; numFracBits "Fraction length:"; OutDataTypeStr "Output data type:"; LastOutDataTypeStr "Last output data type:"
      mask help: Output an identity matrix. If the matrix size entered is a scalar, then the output will be a square (symmetric) identity matrix with the number of rows and columns both equal to the specified value. If the matrix size entered is a two-element vector [M N], then the output will be an asymmetric matrix with the number of rows equal to M, the number of columns equal to N, ones down the diagonal, and zeros elsewhere. This matches the syntax of the MATLAB function eye(N) and eye(M,N), respectively.
      mask init:
      | isCustomFloat =  0; % nice default
      | fxpIsSigned   =  1; % nice default
      | fxpWordLength =  8; % nice default
      | fxpFracLength =  0; % nice default
      | if Inherit
      |     dTypeID   = -3; % SAME_AS_INPUT
      | else
      |     dtRows            = dspblkGetDiscreteImpulseDTRowInfo();
      |     [dtInfo, dTypeID] = dspblkUDTMapperOutDType(gcbh, dtRows{1}, 'dataType', 1.0);
      |     isCustomFloat     = dtInfo.DataTypeIsCustomFloat;
      |     if ~isCustomFloat
      |         fxpIsSigned   = dtInfo.DataTypeIsSigned;
      |         fxpWordLength = dtInfo.DataTypeWordLength;
      |         fxpFracLength = dtInfo.DataTypeFracOrMantBits;
      |     end
      | end
      mask Help: eval('blocksethelp');
      mask Callback Inherit: dspblkeye
      mask TypeOptions dataType: double | single | int8 | uint8 | int16 | uint16 | int32 | uint32 | boolean | Fixed-point | User-defined | Inherit via back propagation
      mask TypeOptions fracBitsMode: Best precision | User-defined
      mask Display:
      | if Inherit
      |     disp('eye( )');
      | else
      |     disp(['eye(' , num2str(get_param(gcbh, 'N')), ')']);
      | end
  Matrix Concatenate : Concatenate  Mode=Multidimensional array  ConcatenateDimension=2
  Matrix Concatenate1 : Concatenate  Mode=Multidimensional array  ConcatenateDimension=2
  Matrix Concatenate2 : Concatenate  Mode=Multidimensional array
  Matrix Multiply2 : Product
  Multiply : Product  Inputs=3
  Transpose2 : Math  Operator=transpose  SaturateOnIntegerOverflow=on
  OMEGA : Outport
  wires:
  Gain/1 -> Transpose2/1
  Constant/1 -> Multiply/2
  omega_magnitude/1 -> Multiply/3
  del_t/1 -> Multiply/1
  Identity Matrix/1 -> Matrix Multiply2/2
  Psi_cross/1 -> Add1/2
  Transpose2/1 -> Matrix Concatenate/2
  Cos/1 -> Matrix Multiply2/1, Matrix Concatenate/1
  Psi_vector/1 -> Matrix Concatenate1/1, Gain/1
  Matrix Concatenate/1 -> Matrix Concatenate2/1
  Matrix Concatenate1/1 -> Matrix Concatenate2/2
  Add1/1 -> Matrix Concatenate1/2
  Matrix Multiply2/1 -> Add1/1
  Multiply/1 -> Cos/1
  Matrix Concatenate2/1 -> OMEGA/1

== system UnitTestDebug/MEKF_lib/Triad/Bypass Triad ==
  quat_old : Inport
  Action Port : ActionPort  ActionType=else
  quat_new : Outport
  wires:
  quat_old/1 -> quat_new/1

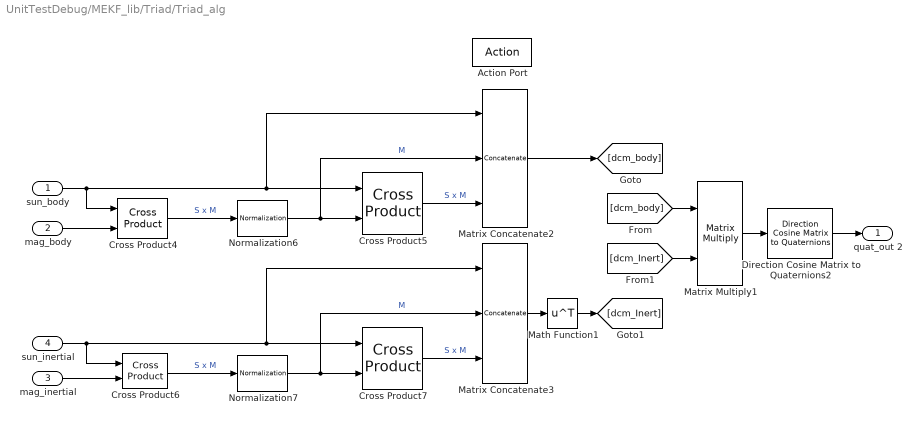
== system UnitTestDebug/MEKF_lib/Triad/Triad_alg ==
  sun_body : Inport
  mag_body : Inport  Port=2
  "mag_inertial " : Inport  Port=3
  sun_inertial : Inport  Port=4
  Action Port : ActionPort  ActionType=then
  Cross Product{4..7} (4 alike) : vrlib/Utilities/Cross Product
      settings: SourceProductBaseCode=VR
  Direction Cosine Matrix to Quaternions2 : sharedtransform/Direction Cosine Matrix  to Quaternions  aMode=0  action=None  tolerance=eps(2)
      settings: SourceProductName=Aerospace Blockset  SourceProductBaseCode=AE
  Math Function1 : Math  Operator=transpose  SaturateOnIntegerOverflow=on
  Matrix Concatenate2 : Concatenate  NumInputs=3  Mode=Multidimensional array  ConcatenateDimension=2
  Matrix Concatenate3 : Concatenate  NumInputs=3  Mode=Multidimensional array  ConcatenateDimension=2
  Matrix Multiply1 : Product  Multiplication=Matrix(*)
  Normalization6 : dspmathops/Normalization  NormType=2-norm  Bias=1e-10  NormOver=Each column  Dimension=1  roundingMode=Floor  overflowMode=off  accumDataTypeStr=Inherit: Same as product output  accumLastDataTypeStr=Inherit: Same as product output  outputDataTypeStr=Inherit: Same as product output  outputMin=[]  outputMax=[]  outputLastDataTypeStr=Inherit: Same as product output
      settings: SourceProductName=DSP System Toolbox
  Normalization7 : dspmathops/Normalization  NormType=2-norm  Bias=1e-10  NormOver=Each column  Dimension=1  roundingMode=Floor  overflowMode=off  accumDataTypeStr=Inherit: Same as product output  accumLastDataTypeStr=Inherit: Same as product output  outputDataTypeStr=Inherit: Same as product output  outputMin=[]  outputMax=[]  outputLastDataTypeStr=Inherit: Same as product output
      settings: SourceProductName=DSP System Toolbox
  quat_out 2 : Outport
  wires:
  [dcm_Inert] -> Matrix Multiply1/2
  [dcm_body] -> Matrix Multiply1/1
  Math Function1/1 -> [dcm_Inert]
  Matrix Concatenate2/1 -> [dcm_body]
  Direction Cosine Matrix to Quaternions2/1 -> quat_out 2/1
  Matrix Multiply1/1 -> Direction Cosine Matrix to Quaternions2/1
  Matrix Concatenate3/1 -> Math Function1/1
  "mag_inertial "/1 -> Cross Product6/2
  Cross Product6/1 -> Normalization7/1  "S x M"
  Normalization7/1 -> Cross Product7/2, Matrix Concatenate3/2  "M"
  Cross Product7/1 -> Matrix Concatenate3/3  "S x M"
  sun_inertial/1 -> Cross Product7/1, Matrix Concatenate3/1, Cross Product6/1
  Cross Product5/1 -> Matrix Concatenate2/3  "S x M"
  Normalization6/1 -> Cross Product5/2, Matrix Concatenate2/2  "M"
  Cross Product4/1 -> Normalization6/1  "S x M"
  mag_body/1 -> Cross Product4/2
  sun_body/1 -> Cross Product4/1, Cross Product5/1, Matrix Concatenate2/1

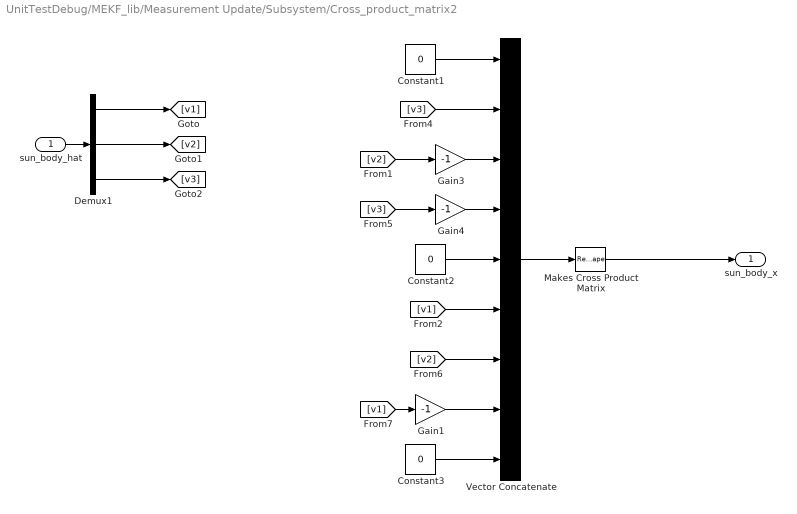
== system UnitTestDebug/MEKF_lib/Measurement Update/Subsystem/Cross_product_matrix2 ==
  sun_body_hat : Inport
  Constant1 : Constant  Value=0
  Constant2 : Constant  Value=0
  Constant3 : Constant  Value=0
  Demux1 : Demux  Outputs=3
  Gain1 : Gain  Gain=-1
  Gain3 : Gain  Gain=-1
  Gain4 : Gain  Gain=-1
  Makes Cross Product Matrix : Reshape  OutputDimensionality=Customize  OutputDimensions=[3,3]
  Vector Concatenate : Concatenate  NumInputs=9
  sun_body_x : Outport
  wires:
  Makes Cross Product Matrix/1 -> sun_body_x/1
  Demux1/1 -> [v1]
  [v1] -> Vector Concatenate/6
  Constant3/1 -> Vector Concatenate/9
  [v3] -> Gain4/1
  Demux1/3 -> [v3]
  Vector Concatenate/1 -> Makes Cross Product Matrix/1
  Constant2/1 -> Vector Concatenate/5
  Demux1/2 -> [v2]
  [v2] -> Vector Concatenate/7
  [v3] -> Vector Concatenate/2
  sun_body_hat/1 -> Demux1/1
  Gain3/1 -> Vector Concatenate/3
  [v1] -> Gain1/1
  Constant1/1 -> Vector Concatenate/1
  [v2] -> Gain3/1
  Gain4/1 -> Vector Concatenate/4
  Gain1/1 -> Vector Concatenate/8

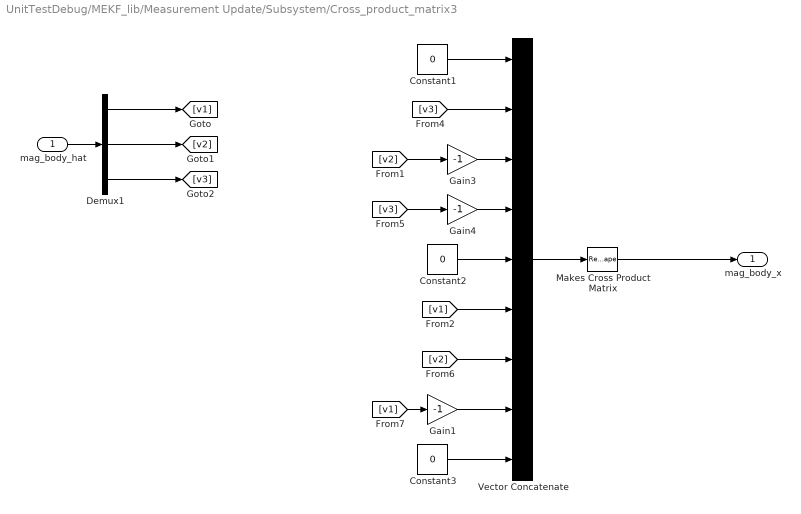
== system UnitTestDebug/MEKF_lib/Measurement Update/Subsystem/Cross_product_matrix3 ==
  mag_body_hat : Inport
  Constant1 : Constant  Value=0
  Constant2 : Constant  Value=0
  Constant3 : Constant  Value=0
  Demux1 : Demux  Outputs=3
  Gain1 : Gain  Gain=-1
  Gain3 : Gain  Gain=-1
  Gain4 : Gain  Gain=-1
  Makes Cross Product Matrix : Reshape  OutputDimensionality=Customize  OutputDimensions=[3,3]
  Vector Concatenate : Concatenate  NumInputs=9
  mag_body_x : Outport
  wires:
  [v2] -> Gain3/1
  Constant3/1 -> Vector Concatenate/9
  Gain4/1 -> Vector Concatenate/4
  Demux1/2 -> [v2]
  Vector Concatenate/1 -> Makes Cross Product Matrix/1
  Constant2/1 -> Vector Concatenate/5
  Demux1/3 -> [v3]
  Makes Cross Product Matrix/1 -> mag_body_x/1
  [v1] -> Gain1/1
  Constant1/1 -> Vector Concatenate/1
  Gain1/1 -> Vector Concatenate/8
  Demux1/1 -> [v1]
  [v3] -> Vector Concatenate/2
  [v3] -> Gain4/1
  Gain3/1 -> Vector Concatenate/3
  [v2] -> Vector Concatenate/7
  [v1] -> Vector Concatenate/6
  mag_body_hat/1 -> Demux1/1

== system UnitTestDebug/MEKF_lib/Time Propagation (q,P)/Psi/If Action Subsystem ==
  del_t : Inport
  omega_vec : Inport  Port=2
  omega_mag : Inport  Port=3
  Action Port : ActionPort  ActionType=else
  Constant : Constant  Value=0.5
  Divide : Product  Inputs=***
  Divide1 : Product  Inputs=**/
  Sin : Trigonometry
  Psi : Outport
  wires:
  Sin/1 -> Divide1/1  "sin(om_mag*0.5*del_t)"
  del_t/1 -> Divide/1
  Divide/1 -> Sin/1
  omega_vec/1 -> Divide1/2
  Constant/1 -> Divide/2
  omega_mag/1 -> Divide/3, Divide1/3
  Divide1/1 -> Psi/1  "Psi"

== system UnitTestDebug/MEKF_lib/Time Propagation (q,P)/Psi/If Action Subsystem1 ==
  Action Port : ActionPort  ActionType=then
  Constant : Constant  Value=0
  Constant1 : Constant  Value=0
  Constant2 : Constant  Value=0
  Mux : Mux  Inputs=3
  Psi_zero : Outport
  wires:
  Mux/1 -> Psi_zero/1
  Constant2/1 -> Mux/3
  Constant1/1 -> Mux/2
  Constant/1 -> Mux/1

== matlab function UnitTestDebug/MATLAB Function ==
  data: v_input input; v_perp output
function v_perp = find_perp(v_input)
%FIND_PERP Finds one of the infinitely number of perpendicular vectors of
%   the input. The input vector v_input is a size 3,1 or 3,1 vector (only
%   3-dim supported)
    
    if length(v_input) ~= 3     % Can't be wrong dim if len=3
        error('find_perp:WrongSize','Input vector has wrong size');
    end
    
    if sum(v_input ~= 0) == 0
        error('find_perp:GivenZeroVector','Zero vector given as input');
    end
    
    v_perp = zeros(size(v_input));
    
    if sum(v_input ~= 0) == 3       % Every element is not-zero
        v_perp(1) = 1;
        v_perp(3) = -v_input(1)/(v_input(3));
    elseif sum(v_input ~= 0) == 2
        if v_input(1) == 0
            v_perp(1:2) = [1 1];
            v_perp(3) = -v_input(2)/(v_input(3));
        elseif v_input(2) == 0
            v_perp(1:2) = [1 1];
            v_perp(3) = -v_input(1)/(v_input(3));
        else
            v_perp(2:3) = [1 1];
            v_perp(1) = -v_input(2)/(v_input(1));
        end
    else
        if v_input(1) ~= 0
            v_perp(2) = 1;
        else
            v_perp(1) = 1;
        end
    end
    
    if abs(dot(v_perp,v_input)) > 1E-09      % Must take round-off into account (the dot product is not always perfect zero)
        error('find_perp:DotProdNotZero',...
            'A perp vector could not be found (failed dot product test). Might there be a bug?');
    end
end

== matlab function UnitTestDebug/MEKF_lib/Time Propagation (q,P)/MATLAB Function1 ==
  data: Phi input; P_plus1 output; Pk_min input; Q_k input
function P_plus1 = fcn(Phi,Pk_min,Q_k)
%#codegen

P_plus1 = Phi*Pk_min*Phi' + Q_k;

== matlab function UnitTestDebug/Subsystem/MATLAB Function ==
  data: v_input input; v_perp output
function v_perp = find_perp(v_input)
%FIND_PERP Finds one of the infinitely number of perpendicular vectors of
%   the input. The input vector v_input is a size 3,1 or 3,1 vector (only
%   3-dim supported)
    
    if length(v_input) ~= 3     % Can't be wrong dim if len=3
        error('find_perp:WrongSize','Input vector has wrong size');
    end
    
    if sum(v_input ~= 0) == 0
        error('find_perp:GivenZeroVector','Zero vector given as input');
    end
    
    v_perp = zeros(size(v_input));
    
    if sum(v_input ~= 0) == 3       % Every element is not-zero
        v_perp(1) = 1;
        v_perp(3) = -v_input(1)/(v_input(3));
    elseif sum(v_input ~= 0) == 2
        if v_input(1) == 0
            v_perp(1:2) = [1 1];
            v_perp(3) = -v_input(2)/(v_input(3));
        elseif v_input(2) == 0
            v_perp(1:2) = [1 1];
            v_perp(3) = -v_input(1)/(v_input(3));
        else
            v_perp(2:3) = [1 1];
            v_perp(1) = -v_input(2)/(v_input(1));
        end
    else
        if v_input(1) ~= 0
            v_perp(2) = 1;
        else
            v_perp(1) = 1;
        end
    end
    
    if abs(dot(v_perp,v_input)) > 1E-09      % Must take round-off into account (the dot product is not always perfect zero)
        error('find_perp:DotProdNotZero',...
            'A perp vector could not be found (failed dot product test). Might there be a bug?');
    end
end
